simulink model "Test1"  (R2017b)
settings: Solver=VariableStepAuto  StartTime=0.0  StopTime=6  MaxStep=1e-4  RelTol=1e-3
libraries: powerlib x13, powerlib_extras x1
settings Model: Creator=80573  LastModifiedBy=80573

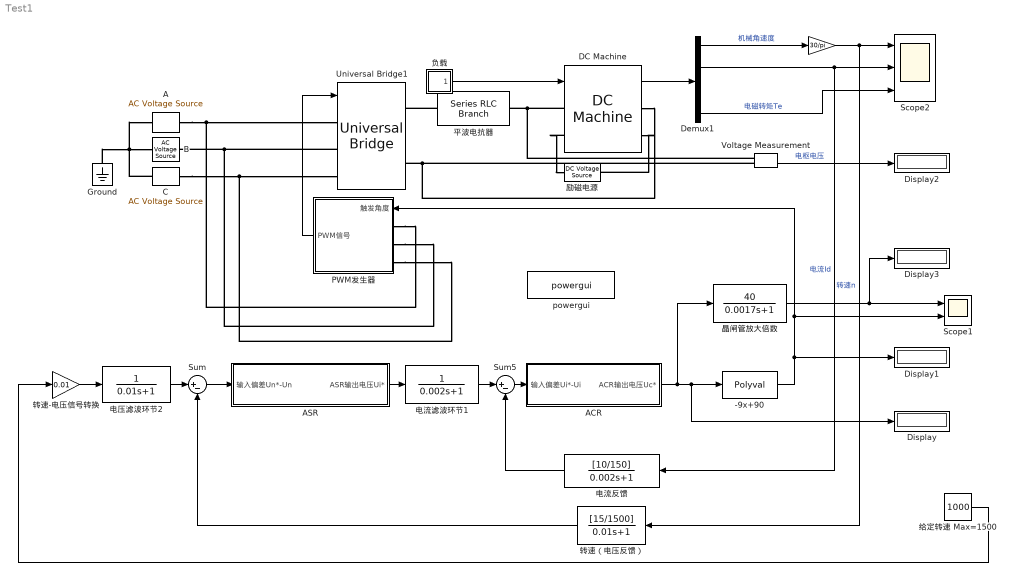
== system Test1 ==
  " " : Gain  Gain=30/pi  SaturateOnIntegerOverflow=on  OutDataTypeStr=Inherit: Same as input  ParamDataTypeStr=Inherit: Same as input
  -9x+90 : Polyval  Coefs=[-9 90]
  A : powerlib/Electrical Sources/AC Voltage Source  Amplitude=510  Phase=0  Frequency=50  SampleTime=0  Measurements=None  BusType=swing  Pref=10e3  Qref=0  Qmin=-inf  Qmax=+inf
  ACR : Subsystem
  ASR : Subsystem
  B : powerlib/Electrical Sources/AC Voltage Source  Amplitude=510  Phase=240  Frequency=50  SampleTime=0  Measurements=None  BusType=swing  Pref=10e3  Qref=0  Qmin=-inf  Qmax=+inf
  C : powerlib/Electrical Sources/AC Voltage Source  Amplitude=510  Phase=120  Frequency=50  SampleTime=0  Measurements=None  BusType=swing  Pref=10e3  Qref=0  Qmin=-inf  Qmax=+inf
  DC Machine : powerlib/Machines/DC Machine  PresetModel=No  MechanicalLoad=Torque TL  FieldType=Wound  ShowDetailedParameters=on  MeasurementBus=off  RLa="[0.16  0.0028]"  RLf=[56.25 0]  Laf=0.404  MachineConstant=Torque constant (N.m/A)  Ke=1.8  Kt=1.8  J=1  Bm=0  Tf=0  w0=0  Ifinit=1  TsPowergui=0  TsBlock=-1
  Demux1 : Demux
  Display{,1..3} (4 alike) : Display
  Ground : powerlib/Elements/Ground  LConnTagsString=a
  PWM发生器 : Subsystem
  Scope1 : Scope  NumInputPorts=2
  Scope2 : Scope  NumInputPorts=3
  Sum : Sum  Inputs=|+-
  Sum5 : Sum  Inputs=|+-
  Universal Bridge1 : powerlib/Power Electronics/Universal Bridge  Arms=3  SnubberResistance=1e5  SnubberCapacitance=inf  Device=Thyristors  Ron=0.5  Lon=0  ForwardVoltages="[  0  0  ]"  ForwardVoltage=0  GTOparameters=[ 10e-6 , 20e-6 ]  IGBTparameters=[ 1e-6 , 2e-6 ]  Measurements=None  Measurements_2=None  converterType=Rectifier
  Voltage Measurement : powerlib/Measurements/Voltage Measurement  PhasorSimulation=off  OutputType=Complex  PSBequivalent=0
  powergui : powerlib/powergui  SimulationMode=Continuous  SampleTime=0.00001  frequency=50  Iterations=50  frequencyindice=0  Pbase=100e6  ErrMax=1e-4  UnitsV=kV  UnitsW=MW  buscounter=0  FunctionMessages=off  echomessages=off  EnableUseOfTLC=off  CurrentSourceSwitches=off  DisableSnubberDevices=off  DisableRonSwitches=off  DisableVfSwitches=off  DisplayEquations=off  SolverType=Tustin/Backward Euler (TBE)  Interpol=off  ExternalGateDelay=off  methode=off  Ts=100  x0status=zero  SPID=on  SwTol=0  HookPort=off  RestoreLinks=warning  ResistiveCurrentMeasurement=off  Frange=[0:2:500]  Ylog=off  Xlog=on  ShowGrid=off  save=off  variable=ZData  structure=0  ZoomFFT=on  StartTime=0.0  cycles=1  DisplayStyle=1  fundamental=60  FreqAxis=off  MaxFrequency=1000  frequencyindicesteady=1  RmsSteady=1  display=off
  励磁电源 : powerlib/Electrical Sources/DC Voltage Source  Amplitude=380  Measurements=None
  平波电抗器 : powerlib/Elements/Series RLC Branch  LConnTagsString=__new0  RConnTagsString=__new0  BranchType=L  Resistance=0.001  Inductance=20e-3  SetiL0=off  InitialCurrent=0  Capacitance=1e-6  Setx0=off  InitialVoltage=0  Measurements=None
  晶闸管放大倍数 : TransferFcn  Numerator=[40]  Denominator=[0.0017 1]
  电压滤波环节2 : TransferFcn  Denominator=[0.01 1]
  电流反馈 : TransferFcn  Numerator=[10/150]  Denominator=[0.002 1]
  电流滤波环节1 : TransferFcn  Denominator=[0.002 1]
  给定转速 Max=1500 : Constant  Value=1000
  负载 : Subsystem
  转速-电压信号转换 : Gain  Gain=0.01
  转速（电压反馈） : TransferFcn  Numerator=[15/1500]  Denominator=[0.01 1]
  wires:
  电流滤波环节1/1 -> Sum5/1
  -9x+90/1 -> Display1/1, Scope1/2, PWM发生器/1(触发角度)
  Voltage Measurement/1 -> Display2/1  "电枢电压"
  Demux1/1 -> " "/1  "机械角速度"
  ACR/1(ACR输出电压Uc*) -> 晶闸管放大倍数/1, Display/1, -9x+90/1
  PWM发生器/1(PWM信号) -> Universal Bridge1/1
  转速-电压信号转换/1 -> 电压滤波环节2/1
  电压滤波环节2/1 -> Sum/1
  电流反馈/1 -> Sum5/2
  " "/1 -> Scope2/1, 转速（电压反馈）/1  "转速n"
  给定转速 Max=1500/1 -> 转速-电压信号转换/1
  转速（电压反馈）/1 -> Sum/2
  Sum5/1 -> ACR/1(输入偏差Ui*-Ui)
  Demux1/2 -> Scope2/2, 电流反馈/1  "电流Id"
  ASR/1(ASR输出电压Ui*) -> 电流滤波环节1/1
  负载/1(TL) -> DC Machine/1
  DC Machine/1 -> Demux1/1
  晶闸管放大倍数/1 -> Scope1/1, Display3/1
  Sum/1 -> ASR/1(输入偏差Un*-Un)
  Demux1/4 -> Scope2/3  "电磁转矩Te"
  connections:
  C/RConn1 -- PWM发生器/LConn3 -- Universal Bridge1/LConn3
  Universal Bridge1/LConn2 -- PWM发生器/LConn2 -- B/RConn1
  C/LConn1 -- B/LConn1 -- Ground/LConn1 -- A/LConn1
  DC Machine/RConn1 -- Voltage Measurement/LConn2 -- Universal Bridge1/RConn2
  A/RConn1 -- PWM发生器/LConn1 -- Universal Bridge1/LConn1
  DC Machine/LConn1 -- Voltage Measurement/LConn1 -- 平波电抗器/RConn1
  平波电抗器/LConn1 -- Universal Bridge1/RConn1
  DC Machine/LConn2 -- 励磁电源/RConn1
  DC Machine/RConn2 -- 励磁电源/LConn1

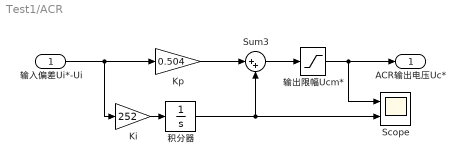
== system Test1/ACR ==
  输入偏差Ui*-Ui : Inport
  Ki : Gain  Gain=252
  Kp : Gain  Gain=0.504
  Scope : Scope  NumInputPorts=2
  Sum3 : Sum  Inputs=|++
  积分器 : Integrator  LimitOutput=on  UpperSaturationLimit=10  LowerSaturationLimit=-12
  输出限幅Ucm* : Saturate  UpperLimit=9  LowerLimit=-10
  ACR输出电压Uc* : Outport
  wires:
  积分器/1 -> Sum3/2, Scope/2
  Ki/1 -> 积分器/1
  Kp/1 -> Sum3/1
  输入偏差Ui*-Ui/1 -> Ki/1, Kp/1
  Sum3/1 -> 输出限幅Ucm*/1
  输出限幅Ucm*/1 -> Scope/1, ACR输出电压Uc*/1

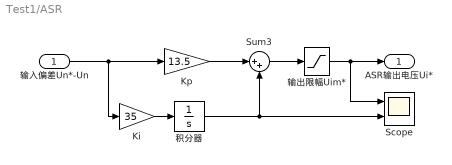
== system Test1/ASR ==
  输入偏差Un*-Un : Inport
  Ki : Gain  Gain=35
  Kp : Gain  Gain=13.5
  Scope : Scope  NumInputPorts=2
  Sum3 : Sum  Inputs=|++
  积分器 : Integrator  LimitOutput=on  UpperSaturationLimit=15  LowerSaturationLimit=-17
  输出限幅Uim* : Saturate  UpperLimit=13  LowerLimit=-15
  ASR输出电压Ui* : Outport
  wires:
  积分器/1 -> Scope/2, Sum3/2
  Ki/1 -> 积分器/1
  Kp/1 -> Sum3/1
  输入偏差Un*-Un/1 -> Ki/1, Kp/1
  Sum3/1 -> 输出限幅Uim*/1
  输出限幅Uim*/1 -> Scope/1, ASR输出电压Ui*/1

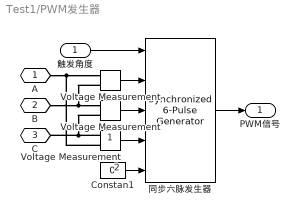
== system Test1/PWM发生器 ==
  触发角度 : Inport
  Constan1 : Constant  Value=0
  Voltage Measurement : powerlib/Measurements/Voltage Measurement  PhasorSimulation=off  OutputType=Complex  PSBequivalent=0
  Voltage Measurement1 : powerlib/Measurements/Voltage Measurement  PhasorSimulation=off  OutputType=Complex  PSBequivalent=0
  Voltage Measurement2 : powerlib/Measurements/Voltage Measurement  PhasorSimulation=off  OutputType=Complex  PSBequivalent=0
  同步六脉发生器 : powerlib_extras/Control  Blocks/Synchronized 6-Pulse Generator  freq=50  pwidth=10  Double_Pulse=on
  A : PMIOPort  Port=1  Side=Left
  B : PMIOPort  Port=2  Side=Left
  C : PMIOPort  Port=3  Side=Left
  PWM信号 : Outport
  wires:
  同步六脉发生器/1 -> PWM信号/1
  Voltage Measurement/1 -> 同步六脉发生器/2
  触发角度/1 -> 同步六脉发生器/1
  Constan1/1 -> 同步六脉发生器/5
  Voltage Measurement1/1 -> 同步六脉发生器/3
  Voltage Measurement2/1 -> 同步六脉发生器/4
  connections:
  A/RConn1 -- Voltage Measurement2/LConn2 -- Voltage Measurement/LConn1
  B/RConn1 -- Voltage Measurement/LConn2 -- Voltage Measurement1/LConn1
  Voltage Measurement2/LConn1 -- Voltage Measurement1/LConn2 -- C/RConn1

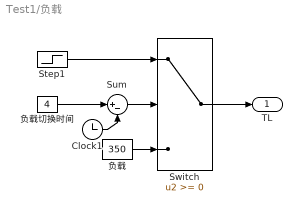
== system Test1/负载 ==
  Clock1 : Clock
  Step1 : Step  Time=2  Before=200  After=500  SampleTime=0
  Sum : Sum  Inputs=|+-
  Switch : Switch
  负载 : Constant  Value=350
  负载切换时间 : Constant  Value=4
  TL : Outport
  wires:
  Clock1/1 -> Sum/2
  Switch/1 -> TL/1
  Sum/1 -> Switch/2
  负载/1 -> Switch/3
  负载切换时间/1 -> Sum/1
  Step1/1 -> Switch/1
